simulink model "ProvaSCADA"  (R2024b)
settings: Solver=FixedStepAuto  StartTime=0.0  StopTime=Tsim  FixedStep=dT  RelTol=1e-3
values from neighbouring files (symbols this model uses):
  b = t + 2*s    (= 3.6)    [ParametriSegheria.m]    (also in ParametriSegheriaDinamica.m)
  h_index = [70, 80, 90, 100]    [ParametriSegheria.m]    (also in ParametriSegheriaDinamica.m)
  J1 = 8*1e6    (= 8000000)    [ParametriSegheriaDinamica.m]
  J2 = 0.9*1e6    (= 900000)    [ParametriSegheriaDinamica.m]
  kc = [0 35 40 50 55 90]    [ParametriSegheria.m]    (also in ParametriSegheriaDinamica.m = [0, 25, 30, 35, 50, 70])
  Kt = 2    [ParametriSegheria.m]    (also in ParametriSegheriaDinamica.m = 10000)
  Kt2 = 5    [ParametriSegheria.m]    (also in ParametriSegheriaDinamica.m = 4500)
  l_index = [20, 30, 40, 50]    [ParametriSegheria.m]    (also in ParametriSegheriaDinamica.m)
  Lt = 4    [ParametriSegheria.m]    (also in ParametriSegheriaDinamica.m)
  Mag_D = [0 430 320 260 230 540 430 320 260 230 540 430 320 260 230 540 430 320 260 230 540 430 320 260 230 540 430 320 260 230 540]    [ParametriSegheria.m]    (also in ParametriSegheriaDinamica.m = [0 randi([220 500], 1, 150)])
  Mag_legno = [0 1 5 2 4 3 1 5 2 4 3 1 5 2 4 3 1 5 2 4 3 1 5 2 4 3 1 5 2 4 3]    [ParametriSegheria.m]    (also in ParametriSegheriaDinamica.m = [0 randi([1 5], 1, 150)])
  n_sottili = 4    [ParametriSegheria.m]    (also in ParametriSegheriaDinamica.m)
  omega_ref1 = 50    [ParametriSegheriaDinamica.m]
  omega_ref2 = 3000*(2*pi/60)    (= 314.159265359)    [ParametriSegheriaDinamica.m]
  Rc = 200    [ParametriSegheria.m]    (also in ParametriSegheriaDinamica.m)
  rho = [0, 450, 520, 590, 710, 780]*1e-9    [ParametriSegheriaDinamica.m]
  Rs = 800    [ParametriSegheria.m]    (also in ParametriSegheriaDinamica.m)
  SR = Rs/Rm    (= 5.33333333333)    [ParametriSegheria.m]    (also in ParametriSegheriaDinamica.m)
  SR2 = Rc/Rm2    (= 4)    [ParametriSegheria.m]    (also in ParametriSegheriaDinamica.m)
undefined symbols (not defined in the file or in its folder): thrsh
libraries: simulink x6, slpidlib x6
(part 1 of 2)
settings Model: Creator=samue  LastModifiedBy=samue

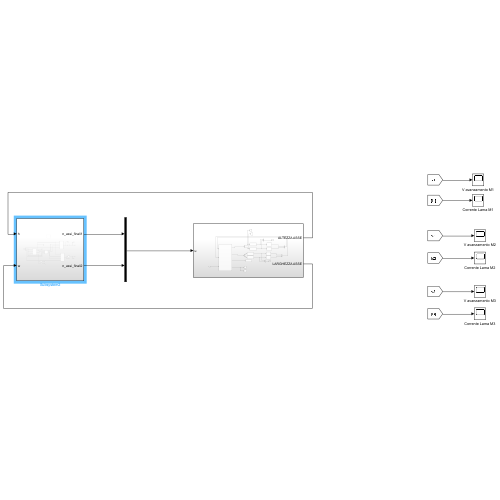
[thumbnail: Simulink's stored preview of the top-level diagram]
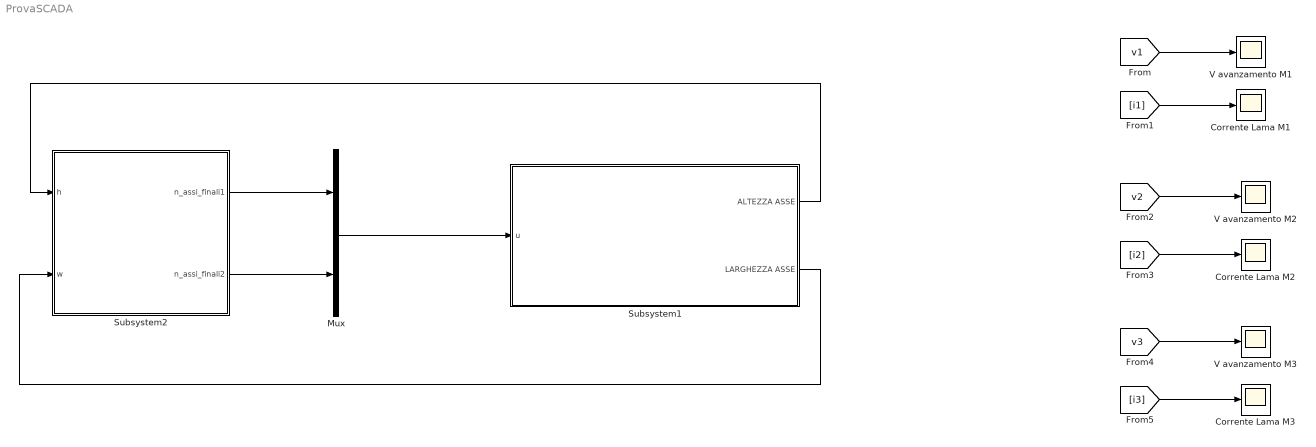
== system ProvaSCADA ==
  Corrente Lama M1 : Scope
  Corrente Lama M2 : Scope
  Corrente Lama M3 : Scope
  Mux : Mux  Inputs=2
  Subsystem1 : Subsystem
  Subsystem2 : Subsystem
  V avanzamento M1 : Scope
  V avanzamento M2 : Scope
  V avanzamento M3 : Scope
  wires:
  Subsystem2/2(n_assi_finali2) -> Mux/2
  [i3] -> Corrente Lama M3/1
  [i1] -> Corrente Lama M1/1
  [i2] -> Corrente Lama M2/1
  Subsystem2/1(n_assi_finali1) -> Mux/1
  [v2] -> V avanzamento M2/1
  [v1] -> V avanzamento M1/1
  [v3] -> V avanzamento M3/1
  Mux/1 -> Subsystem1/1(u)
  Subsystem1/1(ALTEZZA ASSE) -> Subsystem2/1(h)
  Subsystem1/2(LARGHEZZA ASSE) -> Subsystem2/2(w)

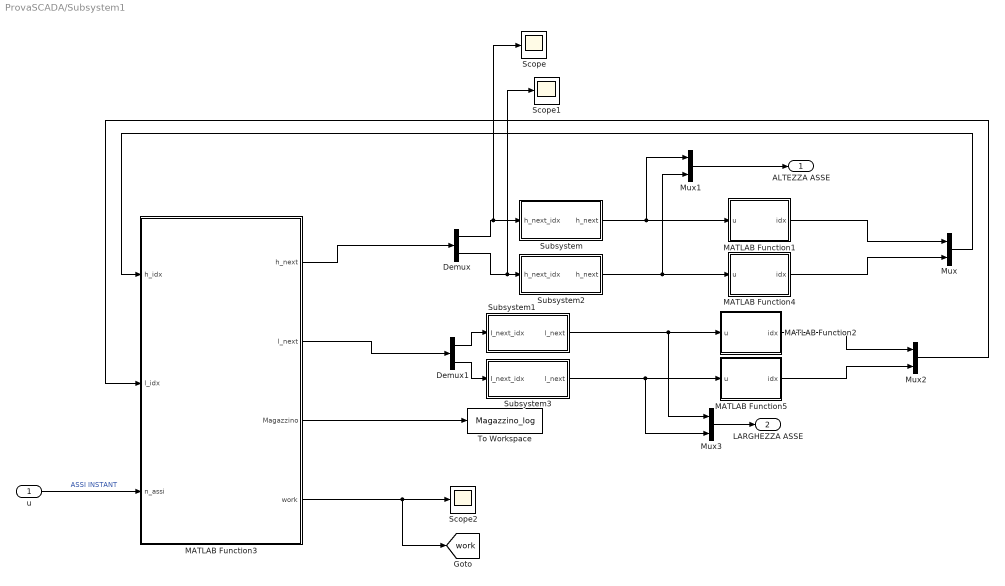
== system ProvaSCADA/Subsystem1 ==
  u : Inport
  Demux : Demux  Outputs=2
  Demux1 : Demux  Outputs=2
  MATLAB Function1 : MATLAB Function  TreatAsAtomicUnit=on
  MATLAB Function2 : MATLAB Function  TreatAsAtomicUnit=on
  MATLAB Function3 : MATLAB Function  TreatAsAtomicUnit=on
  MATLAB Function4 : MATLAB Function  TreatAsAtomicUnit=on
  MATLAB Function5 : MATLAB Function  TreatAsAtomicUnit=on
  Mux{,1..3} (4 alike) : Mux  Inputs=2
  Scope : Scope
  Scope1 : Scope
  Scope2 : Scope
  Subsystem : Subsystem
  Subsystem1 : Subsystem
  Subsystem2 : Subsystem
  Subsystem3 : Subsystem
  To Workspace : ToWorkspace  VariableName=Magazzino_log  SaveFormat=Timeseries  SampleTime=-1
  ALTEZZA ASSE : Outport
  LARGHEZZA ASSE : Outport  Port=2
  tag scope: work=global
  wires:
  MATLAB Function3/3(Magazzino) -> To Workspace/1
  u/1 -> MATLAB Function3/3(n_assi)  "ASSI INSTANT"
  Subsystem/1(h_next) -> Mux1/1, MATLAB Function1/1(u)
  Subsystem1/1(l_next) -> Mux3/1, MATLAB Function2/1(u)
  MATLAB Function3/1(h_next) -> Demux/1
  Subsystem2/1(h_next) -> Mux1/2, MATLAB Function4/1(u)
  Demux/2 -> Scope1/1, Subsystem2/1(h_next_idx)
  Demux/1 -> Scope/1, Subsystem/1(h_next_idx)
  MATLAB Function1/1(idx) -> Mux/1
  MATLAB Function4/1(idx) -> Mux/2
  Mux/1 -> MATLAB Function3/1(h_idx)
  Mux1/1 -> ALTEZZA ASSE/1
  Subsystem3/1(l_next) -> Mux3/2, MATLAB Function5/1(u)
  MATLAB Function3/2(l_next) -> Demux1/1
  Demux1/1 -> Subsystem1/1(I_next_idx)
  Demux1/2 -> Subsystem3/1(I_next_idx)
  Mux3/1 -> LARGHEZZA ASSE/1
  MATLAB Function2/1(idx) -> Mux2/1
  MATLAB Function5/1(idx) -> Mux2/2
  Mux2/1 -> MATLAB Function3/2(l_idx)
  MATLAB Function3/4(work) -> [work], Scope2/1

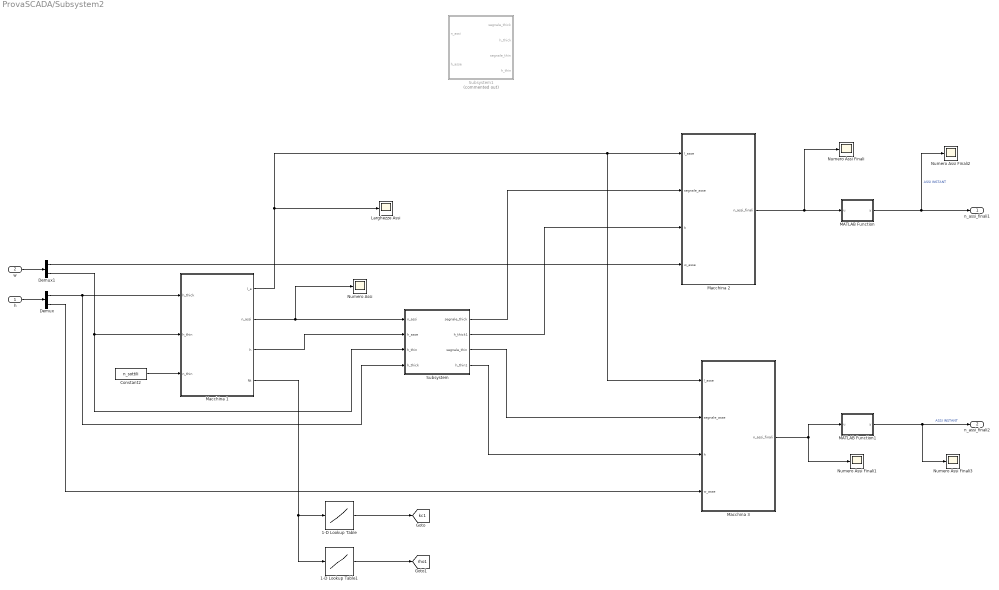
== system ProvaSCADA/Subsystem2 ==
  h : Inport
  w : Inport  Port=2
  1-D Lookup Table : Lookup_n-D  NumberOfTableDimensions=1  BreakpointsForDimension1=[0 1 2 3 4 5 ]  Table=kc  InternalRulePriority=Speed  RndMeth=Simplest
  1-D Lookup Table1 : Lookup_n-D  NumberOfTableDimensions=1  BreakpointsForDimension1=[0 1 2 3 4 5 ]  Table=rho  InternalRulePriority=Speed  RndMeth=Simplest
  Constant2 : Constant  Value=n_sottili
  Demux : Demux  Outputs=2
  Demux1 : Demux  Outputs=2
  Larghezze Assi : Scope
  MATLAB Function : MATLAB Function  TreatAsAtomicUnit=on
  MATLAB Function1 : MATLAB Function  TreatAsAtomicUnit=on
  Macchina 1 : Subsystem
  Macchina 2 : Subsystem
  Macchina 3 : Subsystem
  Numero Assi : Scope
  Numero Assi Finali{,1..3} (4 alike) : Scope
  Subsystem : Subsystem
  Subsystem1 : Subsystem  Commented=on
  n_assi_finali1 : Outport
  n_assi_finali2 : Outport  Port=2
  tag scope: kc1=global, rho1=global
  wires:
  Macchina 1/1(l_a) -> Larghezze Assi/1, Macchina 3/1(l_asse), Macchina 2/1(l_asse)
  Macchina 1/2(n_assi) -> Numero Assi/1, Subsystem/1(n_assi)
  Macchina 1/3(h) -> Subsystem/2(h_asse)
  Constant2/1 -> Macchina 1/3(n_thin)
  Macchina 3/1(n_assi_finali) -> Numero Assi Finali1/1, MATLAB Function1/1(u)
  Macchina 2/1(n_assi_finali) -> Numero Assi Finali/1, MATLAB Function/1(u)
  MATLAB Function/1(y) -> Numero Assi Finali2/1, n_assi_finali1/1  "ASSI INSTANT"
  MATLAB Function1/1(y) -> Numero Assi Finali3/1, n_assi_finali2/1  "ASSI INSTANT"
  Subsystem/1(segnale_thick) -> Macchina 2/2(segnale_asse)
  Subsystem/2(h_thick1) -> Macchina 2/3(h)
  Subsystem/3(segnale_thin) -> Macchina 3/2(segnale_asse)
  Subsystem/4(h_thin1) -> Macchina 3/3(h)
  1-D Lookup Table/1 -> [kc1]
  1-D Lookup Table1/1 -> [rho1]
  Macchina 1/4(Nt) -> 1-D Lookup Table1/1, 1-D Lookup Table/1
  h/1 -> Demux/1
  w/1 -> Demux1/1
  Demux/2 -> Macchina 3/4(w_asse)
  Demux/1 -> Macchina 1/1(h_thick), Subsystem/4(h_thick)
  Demux1/1 -> Macchina 2/4(w_asse)
  Demux1/2 -> Subsystem/3(h_thin), Macchina 1/2(h_thin)

== system ProvaSCADA/Subsystem1/Subsystem ==
  h_next_idx : Inport
  Constant4 : Constant  Value=h_index
  Constant7 : Constant
  Memory : Memory
  SELEZIONE ALTEZZA : Selector  InputPortWidth=length(h_index)  IndexOptions=Index vector (port)  Indices=[1 3]  OutputSizes=1
  Switch1 : Switch  Criteria=u2 > Threshold  SaturateOnIntegerOverflow=off  InputSameDT=off
  h_next : Outport
  wires:
  h_next_idx/1 -> Memory/1
  Constant7/1 -> Switch1/3
  Memory/1 -> Switch1/2, Switch1/1
  SELEZIONE ALTEZZA/1 -> h_next/1
  Constant4/1 -> SELEZIONE ALTEZZA/1
  Switch1/1 -> SELEZIONE ALTEZZA/2

== system ProvaSCADA/Subsystem1/Subsystem1 ==
  I_next_idx : Inport
  Constant5 : Constant  Value=l_index
  Constant8 : Constant
  Memory1 : Memory
  SELEZIONE LUNGHEZZA : Selector  InputPortWidth=length(h_index)  IndexOptions=Index vector (port)  Indices=[1 3]  OutputSizes=1
  Switch2 : Switch  Criteria=u2 > Threshold  SaturateOnIntegerOverflow=off  InputSameDT=off
  l_next : Outport
  wires:
  Memory1/1 -> Switch2/1, Switch2/2
  SELEZIONE LUNGHEZZA/1 -> l_next/1
  Switch2/1 -> SELEZIONE LUNGHEZZA/2
  Constant5/1 -> SELEZIONE LUNGHEZZA/1
  I_next_idx/1 -> Memory1/1
  Constant8/1 -> Switch2/3

== system ProvaSCADA/Subsystem1/Subsystem2 ==
  h_next_idx : Inport
  Constant4 : Constant  Value=h_index
  Constant7 : Constant
  Memory : Memory
  SELEZIONE ALTEZZA : Selector  InputPortWidth=length(h_index)  IndexOptions=Index vector (port)  Indices=[1 3]  OutputSizes=1
  Switch1 : Switch  Criteria=u2 > Threshold  SaturateOnIntegerOverflow=off  InputSameDT=off
  h_next : Outport
  wires:
  Switch1/1 -> SELEZIONE ALTEZZA/2
  Constant4/1 -> SELEZIONE ALTEZZA/1
  SELEZIONE ALTEZZA/1 -> h_next/1
  Memory/1 -> Switch1/1, Switch1/2
  Constant7/1 -> Switch1/3
  h_next_idx/1 -> Memory/1

== system ProvaSCADA/Subsystem1/Subsystem3 ==
  I_next_idx : Inport
  Constant5 : Constant  Value=l_index
  Constant8 : Constant
  Memory1 : Memory
  SELEZIONE LUNGHEZZA : Selector  InputPortWidth=length(h_index)  IndexOptions=Index vector (port)  Indices=[1 3]  OutputSizes=1
  Switch2 : Switch  Criteria=u2 > Threshold  SaturateOnIntegerOverflow=off  InputSameDT=off
  l_next : Outport
  wires:
  Constant8/1 -> Switch2/3
  I_next_idx/1 -> Memory1/1
  Constant5/1 -> SELEZIONE LUNGHEZZA/1
  Switch2/1 -> SELEZIONE LUNGHEZZA/2
  SELEZIONE LUNGHEZZA/1 -> l_next/1
  Memory1/1 -> Switch2/2, Switch2/1

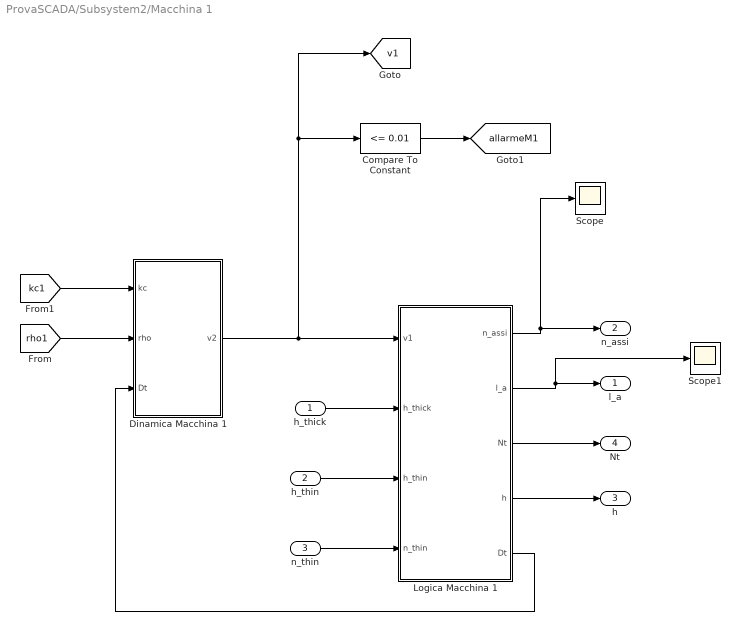
== system ProvaSCADA/Subsystem2/Macchina 1 ==
  h_thick : Inport
  h_thin : Inport  Port=2
  n_thin : Inport  Port=3
  Compare To Constant : simulink/Logic and Bit Operations/Compare To Constant  relop=<=  const=0.01  OutDataTypeStr=boolean
  Dinamica Macchina 1 : Subsystem
  Logica Macchina 1 : Subsystem
  Scope : Scope
  Scope1 : Scope
  l_a : Outport
  n_assi : Outport  Port=2
  h : Outport  Port=3
  Nt : Outport  Port=4
  tag scope: allarmeM1=global, v1=global
  wires:
  Dinamica Macchina 1/1(v2) -> Compare To Constant/1, [v1], Logica Macchina 1/1(v1)
  Logica Macchina 1/3(Nt) -> Nt/1
  Logica Macchina 1/1(n_assi) -> Scope/1, n_assi/1
  Logica Macchina 1/2(l_a) -> Scope1/1, l_a/1
  h_thick/1 -> Logica Macchina 1/2(h_thick)
  h_thin/1 -> Logica Macchina 1/3(h_thin)
  n_thin/1 -> Logica Macchina 1/4(n_thin)
  Logica Macchina 1/4(h) -> h/1
  [rho1] -> Dinamica Macchina 1/2(rho)
  [kc1] -> Dinamica Macchina 1/1(kc)
  Logica Macchina 1/5(Dt) -> Dinamica Macchina 1/3(Dt)
  Compare To Constant/1 -> [allarmeM1]

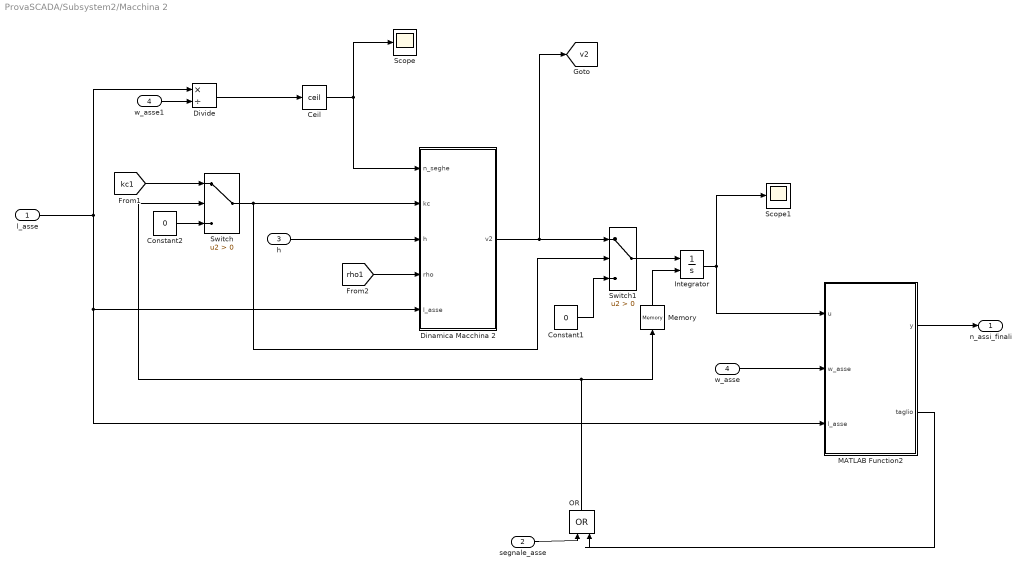
== system ProvaSCADA/Subsystem2/Macchina 2 ==
  l_asse : Inport
  segnale_asse : Inport  Port=2
  h : Inport  Port=3
  w_asse : Inport  Port=4
  Ceil : Rounding  Operator=ceil
  Constant1 : Constant  Value=0
  Constant2 : Constant  Value=0
  Dinamica Macchina 2 : Subsystem
  Divide : Product  Inputs=*/
  Integrator : Integrator  ExternalReset=falling
  MATLAB Function2 : MATLAB Function  TreatAsAtomicUnit=on
  Memory : Memory
  OR : Logic  Operator=OR  IconShape=distinctive  AllPortsSameDT=off  OutDataTypeStr=boolean
  Scope : Scope
  Scope1 : Scope
  Switch : Switch  Criteria=u2 > Threshold  SaturateOnIntegerOverflow=off  InputSameDT=off
  Switch1 : Switch  Criteria=u2 > Threshold  SaturateOnIntegerOverflow=off  InputSameDT=off
  w_asse1 : InportShadow  Port=4
  n_assi_finali : Outport
  tag scope: v2=global
  wires:
  Divide/1 -> Ceil/1
  OR/1 -> Switch/2, Memory/1
  Dinamica Macchina 2/1(v2) -> Switch1/1, [v2]
  Constant2/1 -> Switch/3
  Switch/1 -> Dinamica Macchina 2/2(kc), Switch1/2
  Integrator/1 -> MATLAB Function2/1(u), Scope1/1
  MATLAB Function2/2(taglio) -> OR/2
  h/1 -> Dinamica Macchina 2/3(h)
  l_asse/1 -> MATLAB Function2/3(l_asse), Dinamica Macchina 2/5(l_asse), Divide/1
  Ceil/1 -> Scope/1, Dinamica Macchina 2/1(n_seghe)
  Memory/1 -> Integrator/2
  [kc1] -> Switch/1
  w_asse1/1 -> Divide/2
  segnale_asse/1 -> OR/1
  w_asse/1 -> MATLAB Function2/2(w_asse)
  [rho1] -> Dinamica Macchina 2/4(rho)
  Switch1/1 -> Integrator/1
  Constant1/1 -> Switch1/3
  MATLAB Function2/1(y) -> n_assi_finali/1

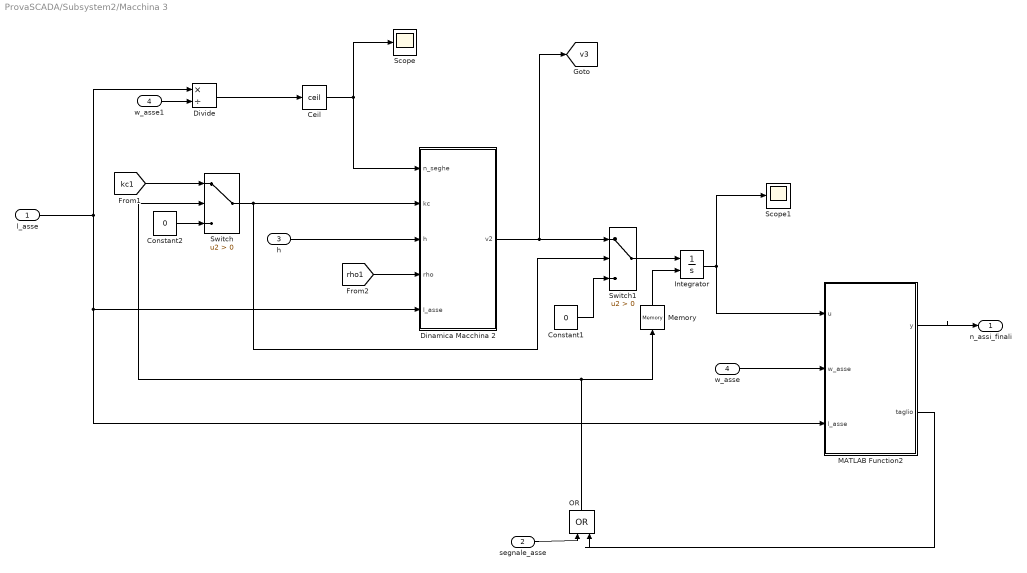
== system ProvaSCADA/Subsystem2/Macchina 3 ==
  l_asse : Inport
  segnale_asse : Inport  Port=2
  h : Inport  Port=3
  w_asse : Inport  Port=4
  Ceil : Rounding  Operator=ceil
  Constant1 : Constant  Value=0
  Constant2 : Constant  Value=0
  Dinamica Macchina 2 : Subsystem
  Divide : Product  Inputs=*/
  Integrator : Integrator  ExternalReset=falling
  MATLAB Function2 : MATLAB Function  TreatAsAtomicUnit=on
  Memory : Memory
  OR : Logic  Operator=OR  IconShape=distinctive  AllPortsSameDT=off  OutDataTypeStr=boolean
  Scope : Scope
  Scope1 : Scope
  Switch : Switch  Criteria=u2 > Threshold  SaturateOnIntegerOverflow=off  InputSameDT=off
  Switch1 : Switch  Criteria=u2 > Threshold  SaturateOnIntegerOverflow=off  InputSameDT=off
  w_asse1 : InportShadow  Port=4
  n_assi_finali : Outport
  tag scope: v3=global
  wires:
  Divide/1 -> Ceil/1
  OR/1 -> Switch/2, Memory/1
  Dinamica Macchina 2/1(v2) -> Switch1/1, [v3]
  Constant2/1 -> Switch/3
  Switch/1 -> Dinamica Macchina 2/2(kc), Switch1/2
  Integrator/1 -> MATLAB Function2/1(u), Scope1/1
  MATLAB Function2/2(taglio) -> OR/2
  h/1 -> Dinamica Macchina 2/3(h)
  l_asse/1 -> MATLAB Function2/3(l_asse), Dinamica Macchina 2/5(l_asse), Divide/1
  Ceil/1 -> Scope/1, Dinamica Macchina 2/1(n_seghe)
  Memory/1 -> Integrator/2
  [kc1] -> Switch/1
  MATLAB Function2/1(y) -> n_assi_finali/1
  w_asse1/1 -> Divide/2
  segnale_asse/1 -> OR/1
  w_asse/1 -> MATLAB Function2/2(w_asse)
  [rho1] -> Dinamica Macchina 2/4(rho)
  Switch1/1 -> Integrator/1
  Constant1/1 -> Switch1/3

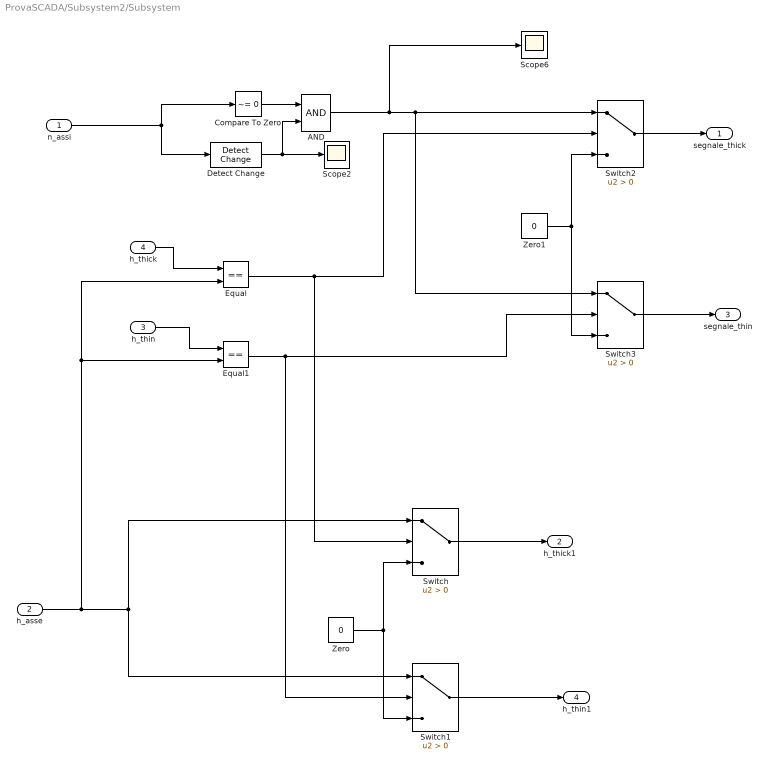
== system ProvaSCADA/Subsystem2/Subsystem ==
  n_assi : Inport
  h_asse : Inport  Port=2
  h_thin : Inport  Port=3
  h_thick : Inport  Port=4
  AND : Logic  IconShape=distinctive  AllPortsSameDT=off  OutDataTypeStr=boolean
  Compare To Zero : simulink/Logic and Bit Operations/Compare To Zero  relop=~=  OutDataTypeStr=boolean
  Detect Change : simulink/Logic and Bit Operations/Detect Change  vinit=0  OutDataTypeStr=boolean
  Equal : RelationalOperator  Operator===  OutDataTypeStr=boolean  RndMeth=Simplest  InputSameDT=off
  Equal1 : RelationalOperator  Operator===  OutDataTypeStr=boolean  RndMeth=Simplest  InputSameDT=off
  Scope2 : Scope
  Scope6 : Scope
  Switch{,1..3} (4 alike) : Switch  Criteria=u2 > Threshold  SaturateOnIntegerOverflow=off  InputSameDT=off
  Zero : Constant  Value=0  OutDataTypeStr=Inherit: Inherit via back propagation
  Zero1 : Constant  Value=0  OutDataTypeStr=Inherit: Inherit via back propagation
  segnale_thick : Outport
  h_thick1 : Outport  Port=2
  segnale_thin : Outport  Port=3
  h_thin1 : Outport  Port=4
  wires:
  Detect Change/1 -> Scope2/1, AND/2
  Zero/1 -> Switch/3, Switch1/3
  Switch/1 -> h_thick1/1
  n_assi/1 -> Compare To Zero/1, Detect Change/1
  Compare To Zero/1 -> AND/1
  Switch1/1 -> h_thin1/1
  Zero1/1 -> Switch2/3, Switch3/3
  h_asse/1 -> Equal1/2, Equal/2, Switch/1, Switch1/1
  Switch2/1 -> segnale_thick/1
  AND/1 -> Switch3/1, Switch2/1, Scope6/1
  Switch3/1 -> segnale_thin/1
  h_thick/1 -> Equal/1
  Equal/1 -> Switch/2, Switch2/2
  h_thin/1 -> Equal1/1
  Equal1/1 -> Switch1/2, Switch3/2

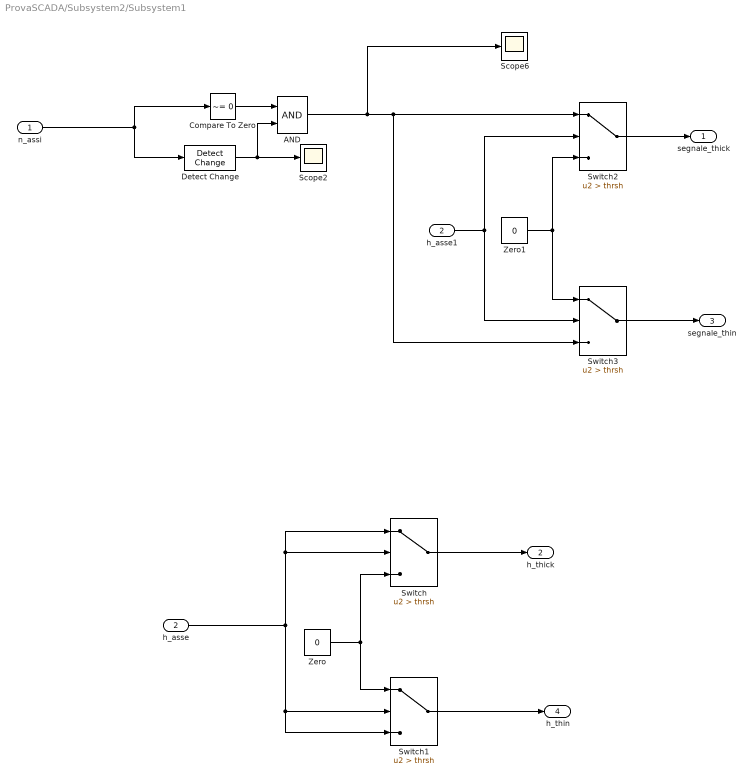
== system ProvaSCADA/Subsystem2/Subsystem1 ==
  n_assi : Inport
  h_asse : Inport  Port=2
  AND : Logic  IconShape=distinctive  AllPortsSameDT=off  OutDataTypeStr=boolean
  Compare To Zero : simulink/Logic and Bit Operations/Compare To Zero  relop=~=  OutDataTypeStr=boolean
  Detect Change : simulink/Logic and Bit Operations/Detect Change  vinit=0  OutDataTypeStr=boolean
  Scope2 : Scope
  Scope6 : Scope
  Switch{,1..3} (4 alike) : Switch  Criteria=u2 > Threshold  Threshold=thrsh  SaturateOnIntegerOverflow=off  InputSameDT=off
  Zero : Constant  Value=0  OutDataTypeStr=Inherit: Inherit via back propagation
  Zero1 : Constant  Value=0  OutDataTypeStr=Inherit: Inherit via back propagation
  h_asse1 : InportShadow  Port=2
  segnale_thick : Outport
  h_thick : Outport  Port=2
  segnale_thin : Outport  Port=3
  h_thin : Outport  Port=4
  wires:
  Detect Change/1 -> Scope2/1, AND/2
  Zero/1 -> Switch1/1, Switch/3
  Switch/1 -> h_thick/1
  n_assi/1 -> Compare To Zero/1, Detect Change/1
  Compare To Zero/1 -> AND/1
  Switch1/1 -> h_thin/1
  Zero1/1 -> Switch2/3, Switch3/1
  h_asse/1 -> Switch/1, Switch/2, Switch1/2, Switch1/3
  Switch2/1 -> segnale_thick/1
  h_asse1/1 -> Switch2/2, Switch3/2
  AND/1 -> Switch3/3, Switch2/1, Scope6/1
  Switch3/1 -> segnale_thin/1

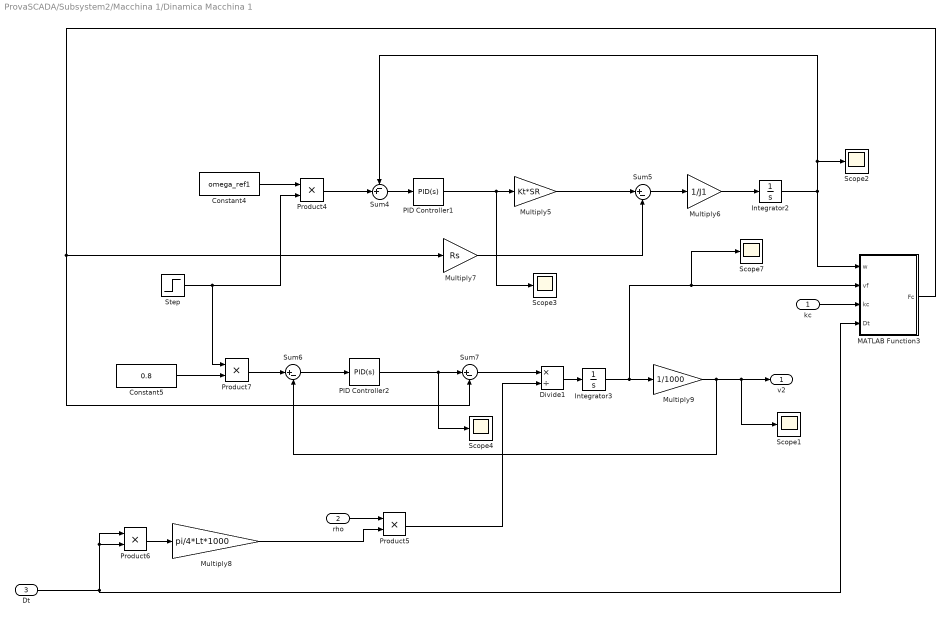
== system ProvaSCADA/Subsystem2/Macchina 1/Dinamica Macchina 1 ==
  kc : Inport
  rho : Inport  Port=2
  Dt : Inport  Port=3
  Constant4 : Constant  Value=omega_ref1
  Constant5 : Constant  Value=0.8
  Divide1 : Product  Inputs=*/
  Integrator2 : Integrator  InitialCondition=omega_ref1
  Integrator3 : Integrator  InitialCondition=800
  MATLAB Function3 : MATLAB Function  TreatAsAtomicUnit=on
  Multiply5 : Gain  Gain=Kt*SR
  Multiply6 : Gain  Gain=1/J1
  Multiply7 : Gain  Gain=Rs
  Multiply8 : Gain  Gain=pi/4*Lt*1000
  Multiply9 : Gain  Gain=1/1000
  PID Controller1 : slpidlib/PID Controller  Controller=PID  Form=Parallel  TimeDomain=Continuous-time  UseExternalTs=off  SampleTime=-1  IntegratorMethod=Forward Euler  FilterMethod=Forward Euler  ControllerParametersSource=internal  P=1298.12673021629  I=2057.42177441043  UseKiTs=off  D=19.7220789716769  UseExternalDerivativeSource=off  N=48.3817350429841  UseFilter=on  TunerSelectOption=Transfer Function Based (PID Tuner App)  InitialConditionSource=internal  InitialConditionForIntegrator=0  InitialConditionForFilter=0  DifferentiatorICPrevScaledInput=0  ExternalReset=none  TrackingMode=off  Kt=1  LimitOutput=on  SatLimitsSource=internal  UpperSaturationLimit=300  LowerSaturationLimit=-300  LinearizeAsGain=off  AntiWindupMode=clamping  Kb=1  LimitIntegrator=off  UpperIntegratorSaturationLimit=200  LowerIntegratorSaturationLimit=-inf  POutMin=[]  POutMax=[]  IOutMin=[]  IOutMax=[]  DOutMin=[]  DOutMax=[]  NOutMin=[]  NOutMax=[]  SumOutMin=[]  SumOutMax=[]  SaturationOutMin=[]  SaturationOutMax=[]  PParamMin=[]  PParamMax=[]  IParamMin=[]  IParamMax=[]  DParamMin=[]  DParamMax=[]  NParamMin=[]  NParamMax=[]  KbParamMin=[]  KbParamMax=[]  KtParamMin=[]  KtParamMax=[]  KbOutMin=[]  KbOutMax=[]  KtOutMin=[]  KtOutMax=[]  IntegratorOutMin=[]  IntegratorOutMax=[]  FilterOutMin=[]  FilterOutMax=[]  SumI1OutMin=[]  SumI1OutMax=[]  SumI2OutMin=[]  SumI2OutMax=[]  SumI3OutMin=[]  SumI3OutMax=[]  SumI4OutMin=[]  SumI4OutMax=[]  SumDOutMin=[]  SumDOutMax=[]  DifferentiatorOutMin=[]  DifferentiatorOutMax=[]  FilterDiffOutCoefMin=[]  FilterDiffOutCoefMax=[]  ReciprocalOutMin=[]  ReciprocalOutMax=[]  SumDenOutMin=[]  SumDenOutMax=[]  SumNumOutMin=[]  SumNumOutMax=[]  DivideOutMin=[]  DivideOutMax=[]  UdiffTsProdOutMin=[]  UdiffTsProdOutMax=[]  NTsProdOutMin=[]  NTsProdOutMax=[]  UintegralTsProdOutMin=[]  UintegralTsProdOutMax=[]  UngainTsProdOutMin=[]  UngainTsProdOutMax=[]  ClampingZeroOutDataTypeStr=Inherit: Inherit via back propagation  ClampingZeroOutMin=[]  ClampingZeroOutMax=[]  FilterDenConstantOutDataTypeStr=Inherit: Inherit via back propagation  FilterDenConstantOutMin=[]  FilterDenConstantOutMax=[]  PCopyOutDataTypeStr=Inherit: Inherit via back propagation  PCopyOutMin=[]  PCopyOutMax=[]  NCopyOutDataTypeStr=Inherit: Inherit via back propagation  NCopyOutMin=[]  NCopyOutMax=[]  IntegratorContinuousStateAttributes=''  IntegratorStateMustResolveToSignalObject=off  IntegratorRTWStateStorageClass=Auto  FilterContinuousStateAttributes=''  FilterStateMustResolveToSignalObject=off  FilterRTWStateStorageClass=Auto  ParallelPVariant=InternalParameters  IdealPVariant=Disabled  IVariant=InternalParameters  DVariant=InternalParameters  IntegratorVariant=Continuous  SatVariant=Enabled  AWVariant=ContClampingParallel  PCopyVariant=Disabled  TRVariant=Disabled  FdbkBlocksVariant=Forward  IdealPFdbkVariant=Disabled  SatFdbkVariant=Disabled  DerivativeFilterVariant=ContFilter  NVariant=InternalParameters  NCopyVariant=Disabled  FilterICVariant=InternalICsFilter  IntegratorICVariant=InternalICs  ExternalResetVariant=Disabled  TRSumVariant=Passthrough  SumFdbkVariant=Disabled  SumVariant=Sum_PID  TsampFilterVariant=InternalTs  TsampNgainVariant=Passthrough  TsampIntegralVariant=Disabled_SignalSpec  ExternalSaturationOutDataTypeStr=Inherit: Same as second input  DerivativeSourceVariant=ErrorSignal  PreIntVariant=InternalPreInt
  PID Controller2 : slpidlib/PID Controller  Controller=PID  Form=Parallel  TimeDomain=Continuous-time  UseExternalTs=off  SampleTime=-1  IntegratorMethod=Forward Euler  FilterMethod=Forward Euler  ControllerParametersSource=internal  P=1286337.49585534  I=1467032.44527875  UseKiTs=off  D=37575.4377581997  UseExternalDerivativeSource=off  N=23.5405770451102  UseFilter=on  TunerSelectOption=Transfer Function Based (PID Tuner App)  InitialConditionSource=internal  InitialConditionForIntegrator=0  InitialConditionForFilter=0  DifferentiatorICPrevScaledInput=0  ExternalReset=none  TrackingMode=off  Kt=1  LimitOutput=on  SatLimitsSource=internal  UpperSaturationLimit=6000  LowerSaturationLimit=-6000  LinearizeAsGain=off  AntiWindupMode=clamping  Kb=1  LimitIntegrator=off  UpperIntegratorSaturationLimit=200  LowerIntegratorSaturationLimit=-inf  POutMin=[]  POutMax=[]  IOutMin=[]  IOutMax=[]  DOutMin=[]  DOutMax=[]  NOutMin=[]  NOutMax=[]  SumOutMin=[]  SumOutMax=[]  SaturationOutMin=[]  SaturationOutMax=[]  PParamMin=[]  PParamMax=[]  IParamMin=[]  IParamMax=[]  DParamMin=[]  DParamMax=[]  NParamMin=[]  NParamMax=[]  KbParamMin=[]  KbParamMax=[]  KtParamMin=[]  KtParamMax=[]  KbOutMin=[]  KbOutMax=[]  KtOutMin=[]  KtOutMax=[]  IntegratorOutMin=[]  IntegratorOutMax=[]  FilterOutMin=[]  FilterOutMax=[]  SumI1OutMin=[]  SumI1OutMax=[]  SumI2OutMin=[]  SumI2OutMax=[]  SumI3OutMin=[]  SumI3OutMax=[]  SumI4OutMin=[]  SumI4OutMax=[]  SumDOutMin=[]  SumDOutMax=[]  DifferentiatorOutMin=[]  DifferentiatorOutMax=[]  FilterDiffOutCoefMin=[]  FilterDiffOutCoefMax=[]  ReciprocalOutMin=[]  ReciprocalOutMax=[]  SumDenOutMin=[]  SumDenOutMax=[]  SumNumOutMin=[]  SumNumOutMax=[]  DivideOutMin=[]  DivideOutMax=[]  UdiffTsProdOutMin=[]  UdiffTsProdOutMax=[]  NTsProdOutMin=[]  NTsProdOutMax=[]  UintegralTsProdOutMin=[]  UintegralTsProdOutMax=[]  UngainTsProdOutMin=[]  UngainTsProdOutMax=[]  ClampingZeroOutDataTypeStr=Inherit: Inherit via back propagation  ClampingZeroOutMin=[]  ClampingZeroOutMax=[]  FilterDenConstantOutDataTypeStr=Inherit: Inherit via back propagation  FilterDenConstantOutMin=[]  FilterDenConstantOutMax=[]  PCopyOutDataTypeStr=Inherit: Inherit via back propagation  PCopyOutMin=[]  PCopyOutMax=[]  NCopyOutDataTypeStr=Inherit: Inherit via back propagation  NCopyOutMin=[]  NCopyOutMax=[]  IntegratorContinuousStateAttributes=''  IntegratorStateMustResolveToSignalObject=off  IntegratorRTWStateStorageClass=Auto  FilterContinuousStateAttributes=''  FilterStateMustResolveToSignalObject=off  FilterRTWStateStorageClass=Auto  ParallelPVariant=InternalParameters  IdealPVariant=Disabled  IVariant=InternalParameters  DVariant=InternalParameters  IntegratorVariant=Continuous  SatVariant=Enabled  AWVariant=ContClampingParallel  PCopyVariant=Disabled  TRVariant=Disabled  FdbkBlocksVariant=Forward  IdealPFdbkVariant=Disabled  SatFdbkVariant=Disabled  DerivativeFilterVariant=ContFilter  NVariant=InternalParameters  NCopyVariant=Disabled  FilterICVariant=InternalICsFilter  IntegratorICVariant=InternalICs  ExternalResetVariant=Disabled  TRSumVariant=Passthrough  SumFdbkVariant=Disabled  SumVariant=Sum_PID  TsampFilterVariant=InternalTs  TsampNgainVariant=Passthrough  TsampIntegralVariant=Disabled_SignalSpec  ExternalSaturationOutDataTypeStr=Inherit: Same as second input  DerivativeSourceVariant=ErrorSignal  PreIntVariant=InternalPreInt
  Product{4..7} (4 alike) : Product
  Scope{1..4,7} (5 alike) : Scope
  Step : Step  Time=5000  Before=1  After=0  SampleTime=0
  Sum4 : Sum  Inputs=-+|
  Sum5 : Sum  Inputs=|+-
  Sum6 : Sum  Inputs=|+-
  Sum7 : Sum  Inputs=|+-
  v2 : Outport
  wires:
  Constant4/1 -> Product4/1
  Constant5/1 -> Product7/2
  Product5/1 -> Divide1/2
  Product4/1 -> Sum4/2
  Sum4/1 -> PID Controller1/1
  Step/1 -> Product4/2, Product7/1
  Product6/1 -> Multiply8/1
  Sum5/1 -> Multiply6/1
  kc/1 -> MATLAB Function3/3(kc)
  Multiply6/1 -> Integrator2/1
  PID Controller1/1 -> Scope3/1, Multiply5/1
  Multiply8/1 -> Product5/2
  MATLAB Function3/1(Fc) -> Sum7/2, Multiply7/1
  Sum6/1 -> PID Controller2/1
  Dt/1 -> Product6/1, Product6/2, MATLAB Function3/4(Dt)
  Divide1/1 -> Integrator3/1
  Integrator3/1 -> Scope7/1, MATLAB Function3/2(vf), Multiply9/1
  Multiply9/1 -> Scope1/1, v2/1, Sum6/2
  Integrator2/1 -> MATLAB Function3/1(w), Scope2/1, Sum4/1
  Sum7/1 -> Divide1/1
  Product7/1 -> Sum6/1
  rho/1 -> Product5/1
  PID Controller2/1 -> Scope4/1, Sum7/1
  Multiply5/1 -> Sum5/1
  Multiply7/1 -> Sum5/2

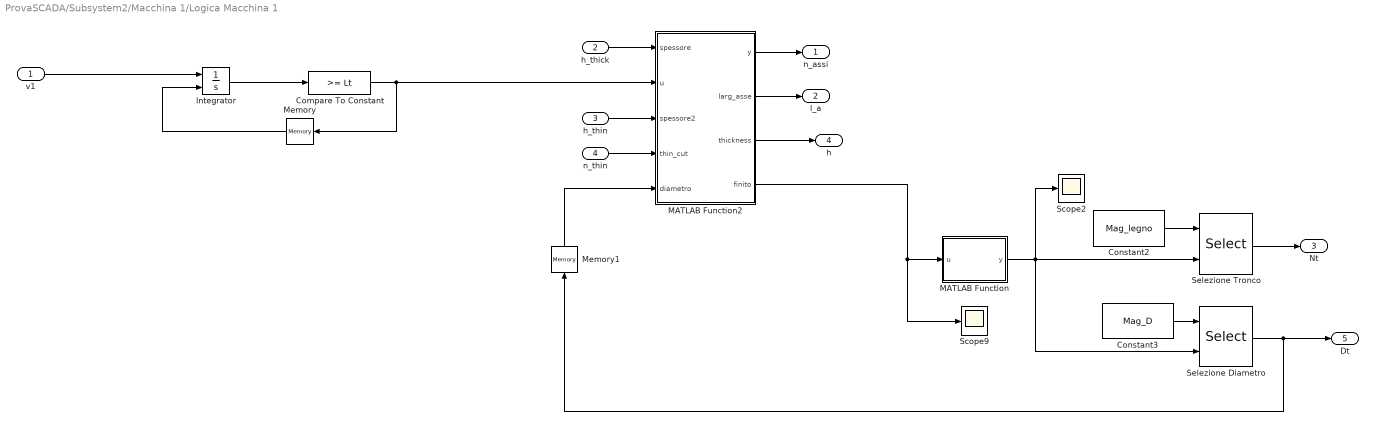
== system ProvaSCADA/Subsystem2/Macchina 1/Logica Macchina 1 ==
  v1 : Inport
  h_thick : Inport  Port=2
  h_thin : Inport  Port=3
  n_thin : Inport  Port=4
  Compare To Constant : simulink/Logic and Bit Operations/Compare To Constant  relop=>=  const=Lt  OutDataTypeStr=boolean
  Constant2 : Constant  Value=Mag_legno
  Constant3 : Constant  Value=Mag_D
  Integrator : Integrator  ExternalReset=rising
  MATLAB Function : MATLAB Function  TreatAsAtomicUnit=on
  MATLAB Function2 : MATLAB Function  TreatAsAtomicUnit=on
  Memory : Memory
  Memory1 : Memory
  Scope2 : Scope
  Scope9 : Scope
  Selezione Diametro : Selector  IndexMode=Zero-based  InputPortWidth=length(Mag_D)  IndexOptions=Index vector (port)  Indices=[1 3]  OutputSizes=1
  Selezione Tronco : Selector  IndexMode=Zero-based  InputPortWidth=length(Mag_legno)  IndexOptions=Index vector (port)  Indices=[1 3]  OutputSizes=1
  n_assi : Outport
  l_a : Outport  Port=2
  Nt : Outport  Port=3
  h : Outport  Port=4
  Dt : Outport  Port=5
  wires:
  Selezione Diametro/1 -> Dt/1, Memory1/1
  MATLAB Function2/4(finito) -> MATLAB Function/1(u), Scope9/1
  Memory/1 -> Integrator/2
  Memory1/1 -> MATLAB Function2/5(diametro)
  Constant2/1 -> Selezione Tronco/1
  v1/1 -> Integrator/1
  Integrator/1 -> Compare To Constant/1
  Constant3/1 -> Selezione Diametro/1
  MATLAB Function/1(y) -> Selezione Diametro/2, Scope2/1, Selezione Tronco/2
  MATLAB Function2/1(y) -> n_assi/1
  Selezione Tronco/1 -> Nt/1
  MATLAB Function2/2(larg_asse) -> l_a/1
  Compare To Constant/1 -> Memory/1, MATLAB Function2/2(u)
  h_thick/1 -> MATLAB Function2/1(spessore)
  h_thin/1 -> MATLAB Function2/3(spessore2)
  n_thin/1 -> MATLAB Function2/4(thin_cut)
  MATLAB Function2/3(thickness) -> h/1

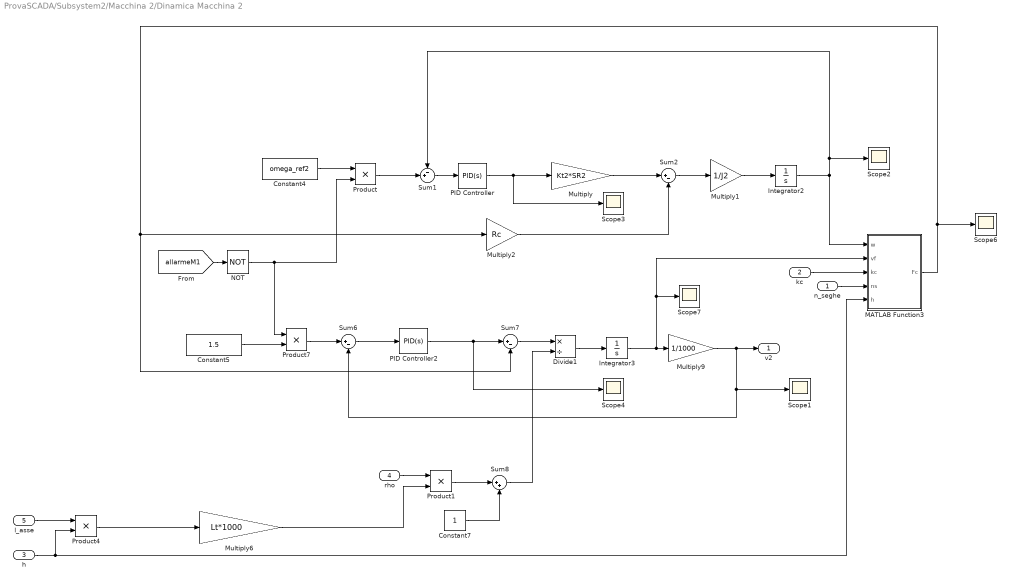
== system ProvaSCADA/Subsystem2/Macchina 2/Dinamica Macchina 2 ==
  n_seghe : Inport
  kc : Inport  Port=2
  h : Inport  Port=3
  rho : Inport  Port=4
  l_asse : Inport  Port=5
  Constant4 : Constant  Value=omega_ref2
  Constant5 : Constant  Value=1.5
  Constant7 : Constant
  Divide1 : Product  Inputs=*/
  Integrator2 : Integrator  InitialCondition=omega_ref2
  Integrator3 : Integrator  InitialCondition=1500
  MATLAB Function3 : MATLAB Function  TreatAsAtomicUnit=on
  Multiply : Gain  Gain=Kt2*SR2
  Multiply1 : Gain  Gain=1/J2
  Multiply2 : Gain  Gain=Rc
  Multiply6 : Gain  Gain=Lt*1000
  Multiply9 : Gain  Gain=1/1000
  NOT : Logic  Operator=NOT  IconShape=distinctive  AllPortsSameDT=off  OutDataTypeStr=boolean
  PID Controller : slpidlib/PID Controller  Controller=PID  Form=Parallel  TimeDomain=Continuous-time  UseExternalTs=off  SampleTime=-1  IntegratorMethod=Forward Euler  FilterMethod=Forward Euler  ControllerParametersSource=internal  P=345.484777327525  I=442.07289174245  UseKiTs=off  D=9.05690517196235  UseExternalDerivativeSource=off  N=26.4189049403583  UseFilter=on  TunerSelectOption=Transfer Function Based (PID Tuner App)  InitialConditionSource=internal  InitialConditionForIntegrator=0  InitialConditionForFilter=0  DifferentiatorICPrevScaledInput=0  ExternalReset=none  TrackingMode=off  Kt=1  LimitOutput=on  SatLimitsSource=internal  UpperSaturationLimit=300  LowerSaturationLimit=-300  LinearizeAsGain=on  AntiWindupMode=clamping  Kb=1  LimitIntegrator=off  UpperIntegratorSaturationLimit=200  LowerIntegratorSaturationLimit=-inf  POutMin=[]  POutMax=[]  IOutMin=[]  IOutMax=[]  DOutMin=[]  DOutMax=[]  NOutMin=[]  NOutMax=[]  SumOutMin=[]  SumOutMax=[]  SaturationOutMin=[]  SaturationOutMax=[]  PParamMin=[]  PParamMax=[]  IParamMin=[]  IParamMax=[]  DParamMin=[]  DParamMax=[]  NParamMin=[]  NParamMax=[]  KbParamMin=[]  KbParamMax=[]  KtParamMin=[]  KtParamMax=[]  KbOutMin=[]  KbOutMax=[]  KtOutMin=[]  KtOutMax=[]  IntegratorOutMin=[]  IntegratorOutMax=[]  FilterOutMin=[]  FilterOutMax=[]  SumI1OutMin=[]  SumI1OutMax=[]  SumI2OutMin=[]  SumI2OutMax=[]  SumI3OutMin=[]  SumI3OutMax=[]  SumI4OutMin=[]  SumI4OutMax=[]  SumDOutMin=[]  SumDOutMax=[]  DifferentiatorOutMin=[]  DifferentiatorOutMax=[]  FilterDiffOutCoefMin=[]  FilterDiffOutCoefMax=[]  ReciprocalOutMin=[]  ReciprocalOutMax=[]  SumDenOutMin=[]  SumDenOutMax=[]  SumNumOutMin=[]  SumNumOutMax=[]  DivideOutMin=[]  DivideOutMax=[]  UdiffTsProdOutMin=[]  UdiffTsProdOutMax=[]  NTsProdOutMin=[]  NTsProdOutMax=[]  UintegralTsProdOutMin=[]  UintegralTsProdOutMax=[]  UngainTsProdOutMin=[]  UngainTsProdOutMax=[]  ClampingZeroOutDataTypeStr=Inherit: Inherit via back propagation  ClampingZeroOutMin=[]  ClampingZeroOutMax=[]  FilterDenConstantOutDataTypeStr=Inherit: Inherit via back propagation  FilterDenConstantOutMin=[]  FilterDenConstantOutMax=[]  PCopyOutDataTypeStr=Inherit: Inherit via back propagation  PCopyOutMin=[]  PCopyOutMax=[]  NCopyOutDataTypeStr=Inherit: Inherit via back propagation  NCopyOutMin=[]  NCopyOutMax=[]  IntegratorContinuousStateAttributes=''  IntegratorStateMustResolveToSignalObject=off  IntegratorRTWStateStorageClass=Auto  FilterContinuousStateAttributes=''  FilterStateMustResolveToSignalObject=off  FilterRTWStateStorageClass=Auto  ParallelPVariant=InternalParameters  IdealPVariant=Disabled  IVariant=InternalParameters  DVariant=InternalParameters  IntegratorVariant=Continuous  SatVariant=Enabled  AWVariant=ContClampingParallel  PCopyVariant=Disabled  TRVariant=Disabled  FdbkBlocksVariant=Forward  IdealPFdbkVariant=Disabled  SatFdbkVariant=Disabled  DerivativeFilterVariant=ContFilter  NVariant=InternalParameters  NCopyVariant=Disabled  FilterICVariant=InternalICsFilter  IntegratorICVariant=InternalICs  ExternalResetVariant=Disabled  TRSumVariant=Passthrough  SumFdbkVariant=Disabled  SumVariant=Sum_PID  TsampFilterVariant=InternalTs  TsampNgainVariant=Passthrough  TsampIntegralVariant=Disabled_SignalSpec  ExternalSaturationOutDataTypeStr=Inherit: Same as second input  DerivativeSourceVariant=ErrorSignal  PreIntVariant=InternalPreInt
  PID Controller2 : slpidlib/PID Controller  Controller=PID  Form=Parallel  TimeDomain=Continuous-time  UseExternalTs=off  SampleTime=-1  IntegratorMethod=Forward Euler  FilterMethod=Forward Euler  ControllerParametersSource=internal  P=20866.9469532593  I=80635.0538109051  UseKiTs=off  D=181.138103439247  UseExternalDerivativeSource=off  N=79.7838174257724  UseFilter=on  TunerSelectOption=Transfer Function Based (PID Tuner App)  InitialConditionSource=internal  InitialConditionForIntegrator=0  InitialConditionForFilter=0  DifferentiatorICPrevScaledInput=0  ExternalReset=none  TrackingMode=off  Kt=1  LimitOutput=on  SatLimitsSource=internal  UpperSaturationLimit=5000  LowerSaturationLimit=-5000  LinearizeAsGain=off  AntiWindupMode=clamping  Kb=1  LimitIntegrator=off  UpperIntegratorSaturationLimit=200  LowerIntegratorSaturationLimit=-inf  POutMin=[]  POutMax=[]  IOutMin=[]  IOutMax=[]  DOutMin=[]  DOutMax=[]  NOutMin=[]  NOutMax=[]  SumOutMin=[]  SumOutMax=[]  SaturationOutMin=[]  SaturationOutMax=[]  PParamMin=[]  PParamMax=[]  IParamMin=[]  IParamMax=[]  DParamMin=[]  DParamMax=[]  NParamMin=[]  NParamMax=[]  KbParamMin=[]  KbParamMax=[]  KtParamMin=[]  KtParamMax=[]  KbOutMin=[]  KbOutMax=[]  KtOutMin=[]  KtOutMax=[]  IntegratorOutMin=[]  IntegratorOutMax=[]  FilterOutMin=[]  FilterOutMax=[]  SumI1OutMin=[]  SumI1OutMax=[]  SumI2OutMin=[]  SumI2OutMax=[]  SumI3OutMin=[]  SumI3OutMax=[]  SumI4OutMin=[]  SumI4OutMax=[]  SumDOutMin=[]  SumDOutMax=[]  DifferentiatorOutMin=[]  DifferentiatorOutMax=[]  FilterDiffOutCoefMin=[]  FilterDiffOutCoefMax=[]  ReciprocalOutMin=[]  ReciprocalOutMax=[]  SumDenOutMin=[]  SumDenOutMax=[]  SumNumOutMin=[]  SumNumOutMax=[]  DivideOutMin=[]  DivideOutMax=[]  UdiffTsProdOutMin=[]  UdiffTsProdOutMax=[]  NTsProdOutMin=[]  NTsProdOutMax=[]  UintegralTsProdOutMin=[]  UintegralTsProdOutMax=[]  UngainTsProdOutMin=[]  UngainTsProdOutMax=[]  ClampingZeroOutDataTypeStr=Inherit: Inherit via back propagation  ClampingZeroOutMin=[]  ClampingZeroOutMax=[]  FilterDenConstantOutDataTypeStr=Inherit: Inherit via back propagation  FilterDenConstantOutMin=[]  FilterDenConstantOutMax=[]  PCopyOutDataTypeStr=Inherit: Inherit via back propagation  PCopyOutMin=[]  PCopyOutMax=[]  NCopyOutDataTypeStr=Inherit: Inherit via back propagation  NCopyOutMin=[]  NCopyOutMax=[]  IntegratorContinuousStateAttributes=''  IntegratorStateMustResolveToSignalObject=off  IntegratorRTWStateStorageClass=Auto  FilterContinuousStateAttributes=''  FilterStateMustResolveToSignalObject=off  FilterRTWStateStorageClass=Auto  ParallelPVariant=InternalParameters  IdealPVariant=Disabled  IVariant=InternalParameters  DVariant=InternalParameters  IntegratorVariant=Continuous  SatVariant=Enabled  AWVariant=ContClampingParallel  PCopyVariant=Disabled  TRVariant=Disabled  FdbkBlocksVariant=Forward  IdealPFdbkVariant=Disabled  SatFdbkVariant=Disabled  DerivativeFilterVariant=ContFilter  NVariant=InternalParameters  NCopyVariant=Disabled  FilterICVariant=InternalICsFilter  IntegratorICVariant=InternalICs  ExternalResetVariant=Disabled  TRSumVariant=Passthrough  SumFdbkVariant=Disabled  SumVariant=Sum_PID  TsampFilterVariant=InternalTs  TsampNgainVariant=Passthrough  TsampIntegralVariant=Disabled_SignalSpec  ExternalSaturationOutDataTypeStr=Inherit: Same as second input  DerivativeSourceVariant=ErrorSignal  PreIntVariant=InternalPreInt
  Product{,1,4,7} (4 alike) : Product
  Scope{1..4,6..7} (6 alike) : Scope
  Sum1 : Sum  Inputs=-+|
  Sum2 : Sum  Inputs=|+-
  Sum6 : Sum  Inputs=|+-
  Sum7 : Sum  Inputs=|+-
  Sum8 : Sum  Inputs=|++
  v2 : Outport
  wires:
  Product4/1 -> Multiply6/1
  h/1 -> MATLAB Function3/5(h), Product4/2
  l_asse/1 -> Product4/1
  Constant4/1 -> Product/1
  Constant5/1 -> Product7/2
  Product/1 -> Sum1/2
  Sum1/1 -> PID Controller/1
  rho/1 -> Product1/1
  NOT/1 -> Product/2, Product7/1
  Multiply1/1 -> Integrator2/1
  PID Controller/1 -> Scope3/1, Multiply/1
  MATLAB Function3/1(Fc) -> Multiply2/1, Sum7/2, Scope6/1
  Sum6/1 -> PID Controller2/1
  Divide1/1 -> Integrator3/1
  Integrator3/1 -> Scope7/1, MATLAB Function3/2(vf), Multiply9/1
  PID Controller2/1 -> Sum7/1, Scope4/1
  Integrator2/1 -> MATLAB Function3/1(w), Scope2/1, Sum1/1
  Sum7/1 -> Divide1/1
  Product7/1 -> Sum6/1
  kc/1 -> MATLAB Function3/3(kc)
  Multiply6/1 -> Product1/2
  n_seghe/1 -> MATLAB Function3/4(ns)
  Product1/1 -> Sum8/1
  Sum8/1 -> Divide1/2
  Constant7/1 -> Sum8/2
  Multiply9/1 -> v2/1, Scope1/1, Sum6/2
  [allarmeM1] -> NOT/1
  Multiply/1 -> Sum2/1
  Sum2/1 -> Multiply1/1
  Multiply2/1 -> Sum2/2

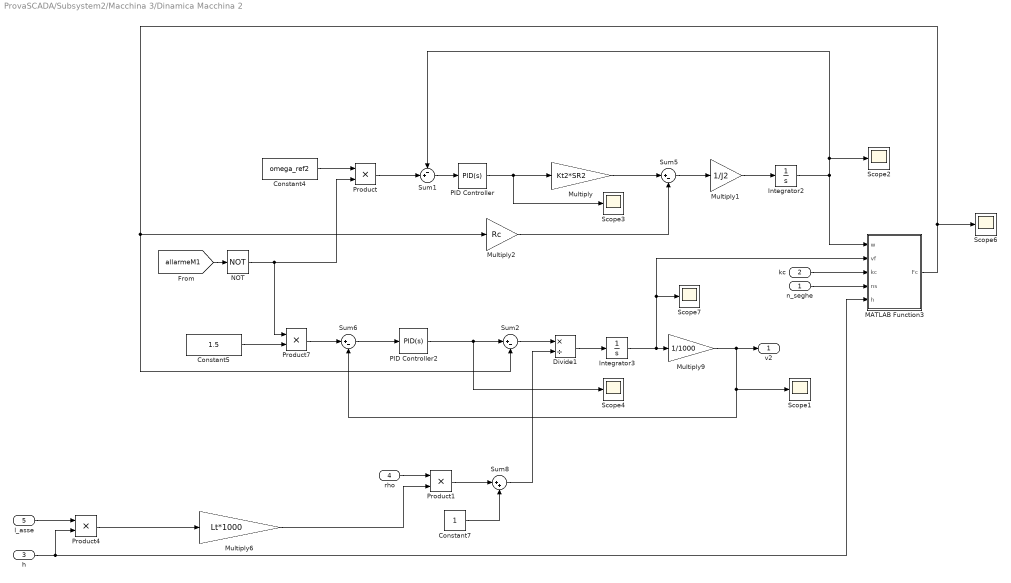
== system ProvaSCADA/Subsystem2/Macchina 3/Dinamica Macchina 2 ==
  n_seghe : Inport
  kc : Inport  Port=2
  h : Inport  Port=3
  rho : Inport  Port=4
  l_asse : Inport  Port=5
  Constant4 : Constant  Value=omega_ref2
  Constant5 : Constant  Value=1.5
  Constant7 : Constant
  Divide1 : Product  Inputs=*/
  Integrator2 : Integrator  InitialCondition=omega_ref2
  Integrator3 : Integrator  InitialCondition=1500
  MATLAB Function3 : MATLAB Function  TreatAsAtomicUnit=on
  Multiply : Gain  Gain=Kt2*SR2
  Multiply1 : Gain  Gain=1/J2
  Multiply2 : Gain  Gain=Rc
  Multiply6 : Gain  Gain=Lt*1000
  Multiply9 : Gain  Gain=1/1000
  NOT : Logic  Operator=NOT  IconShape=distinctive  AllPortsSameDT=off  OutDataTypeStr=boolean
  PID Controller : slpidlib/PID Controller  Controller=PID  Form=Parallel  TimeDomain=Continuous-time  UseExternalTs=off  SampleTime=-1  IntegratorMethod=Forward Euler  FilterMethod=Forward Euler  ControllerParametersSource=internal  P=345.484777327525  I=442.07289174245  UseKiTs=off  D=9.05690517196235  UseExternalDerivativeSource=off  N=26.4189049403583  UseFilter=on  TunerSelectOption=Transfer Function Based (PID Tuner App)  InitialConditionSource=internal  InitialConditionForIntegrator=0  InitialConditionForFilter=0  DifferentiatorICPrevScaledInput=0  ExternalReset=none  TrackingMode=off  Kt=1  LimitOutput=on  SatLimitsSource=internal  UpperSaturationLimit=300  LowerSaturationLimit=-300  LinearizeAsGain=on  AntiWindupMode=clamping  Kb=1  LimitIntegrator=off  UpperIntegratorSaturationLimit=200  LowerIntegratorSaturationLimit=-inf  POutMin=[]  POutMax=[]  IOutMin=[]  IOutMax=[]  DOutMin=[]  DOutMax=[]  NOutMin=[]  NOutMax=[]  SumOutMin=[]  SumOutMax=[]  SaturationOutMin=[]  SaturationOutMax=[]  PParamMin=[]  PParamMax=[]  IParamMin=[]  IParamMax=[]  DParamMin=[]  DParamMax=[]  NParamMin=[]  NParamMax=[]  KbParamMin=[]  KbParamMax=[]  KtParamMin=[]  KtParamMax=[]  KbOutMin=[]  KbOutMax=[]  KtOutMin=[]  KtOutMax=[]  IntegratorOutMin=[]  IntegratorOutMax=[]  FilterOutMin=[]  FilterOutMax=[]  SumI1OutMin=[]  SumI1OutMax=[]  SumI2OutMin=[]  SumI2OutMax=[]  SumI3OutMin=[]  SumI3OutMax=[]  SumI4OutMin=[]  SumI4OutMax=[]  SumDOutMin=[]  SumDOutMax=[]  DifferentiatorOutMin=[]  DifferentiatorOutMax=[]  FilterDiffOutCoefMin=[]  FilterDiffOutCoefMax=[]  ReciprocalOutMin=[]  ReciprocalOutMax=[]  SumDenOutMin=[]  SumDenOutMax=[]  SumNumOutMin=[]  SumNumOutMax=[]  DivideOutMin=[]  DivideOutMax=[]  UdiffTsProdOutMin=[]  UdiffTsProdOutMax=[]  NTsProdOutMin=[]  NTsProdOutMax=[]  UintegralTsProdOutMin=[]  UintegralTsProdOutMax=[]  UngainTsProdOutMin=[]  UngainTsProdOutMax=[]  ClampingZeroOutDataTypeStr=Inherit: Inherit via back propagation  ClampingZeroOutMin=[]  ClampingZeroOutMax=[]  FilterDenConstantOutDataTypeStr=Inherit: Inherit via back propagation  FilterDenConstantOutMin=[]  FilterDenConstantOutMax=[]  PCopyOutDataTypeStr=Inherit: Inherit via back propagation  PCopyOutMin=[]  PCopyOutMax=[]  NCopyOutDataTypeStr=Inherit: Inherit via back propagation  NCopyOutMin=[]  NCopyOutMax=[]  IntegratorContinuousStateAttributes=''  IntegratorStateMustResolveToSignalObject=off  IntegratorRTWStateStorageClass=Auto  FilterContinuousStateAttributes=''  FilterStateMustResolveToSignalObject=off  FilterRTWStateStorageClass=Auto  ParallelPVariant=InternalParameters  IdealPVariant=Disabled  IVariant=InternalParameters  DVariant=InternalParameters  IntegratorVariant=Continuous  SatVariant=Enabled  AWVariant=ContClampingParallel  PCopyVariant=Disabled  TRVariant=Disabled  FdbkBlocksVariant=Forward  IdealPFdbkVariant=Disabled  SatFdbkVariant=Disabled  DerivativeFilterVariant=ContFilter  NVariant=InternalParameters  NCopyVariant=Disabled  FilterICVariant=InternalICsFilter  IntegratorICVariant=InternalICs  ExternalResetVariant=Disabled  TRSumVariant=Passthrough  SumFdbkVariant=Disabled  SumVariant=Sum_PID  TsampFilterVariant=InternalTs  TsampNgainVariant=Passthrough  TsampIntegralVariant=Disabled_SignalSpec  ExternalSaturationOutDataTypeStr=Inherit: Same as second input  DerivativeSourceVariant=ErrorSignal  PreIntVariant=InternalPreInt
  PID Controller2 : slpidlib/PID Controller  Controller=PID  Form=Parallel  TimeDomain=Continuous-time  UseExternalTs=off  SampleTime=-1  IntegratorMethod=Forward Euler  FilterMethod=Forward Euler  ControllerParametersSource=internal  P=20866.9469532593  I=80635.0538109051  UseKiTs=off  D=181.138103439247  UseExternalDerivativeSource=off  N=79.7838174257724  UseFilter=on  TunerSelectOption=Transfer Function Based (PID Tuner App)  InitialConditionSource=internal  InitialConditionForIntegrator=0  InitialConditionForFilter=0  DifferentiatorICPrevScaledInput=0  ExternalReset=none  TrackingMode=off  Kt=1  LimitOutput=on  SatLimitsSource=internal  UpperSaturationLimit=5000  LowerSaturationLimit=-5000  LinearizeAsGain=off  AntiWindupMode=clamping  Kb=1  LimitIntegrator=off  UpperIntegratorSaturationLimit=200  LowerIntegratorSaturationLimit=-inf  POutMin=[]  POutMax=[]  IOutMin=[]  IOutMax=[]  DOutMin=[]  DOutMax=[]  NOutMin=[]  NOutMax=[]  SumOutMin=[]  SumOutMax=[]  SaturationOutMin=[]  SaturationOutMax=[]  PParamMin=[]  PParamMax=[]  IParamMin=[]  IParamMax=[]  DParamMin=[]  DParamMax=[]  NParamMin=[]  NParamMax=[]  KbParamMin=[]  KbParamMax=[]  KtParamMin=[]  KtParamMax=[]  KbOutMin=[]  KbOutMax=[]  KtOutMin=[]  KtOutMax=[]  IntegratorOutMin=[]  IntegratorOutMax=[]  FilterOutMin=[]  FilterOutMax=[]  SumI1OutMin=[]  SumI1OutMax=[]  SumI2OutMin=[]  SumI2OutMax=[]  SumI3OutMin=[]  SumI3OutMax=[]  SumI4OutMin=[]  SumI4OutMax=[]  SumDOutMin=[]  SumDOutMax=[]  DifferentiatorOutMin=[]  DifferentiatorOutMax=[]  FilterDiffOutCoefMin=[]  FilterDiffOutCoefMax=[]  ReciprocalOutMin=[]  ReciprocalOutMax=[]  SumDenOutMin=[]  SumDenOutMax=[]  SumNumOutMin=[]  SumNumOutMax=[]  DivideOutMin=[]  DivideOutMax=[]  UdiffTsProdOutMin=[]  UdiffTsProdOutMax=[]  NTsProdOutMin=[]  NTsProdOutMax=[]  UintegralTsProdOutMin=[]  UintegralTsProdOutMax=[]  UngainTsProdOutMin=[]  UngainTsProdOutMax=[]  ClampingZeroOutDataTypeStr=Inherit: Inherit via back propagation  ClampingZeroOutMin=[]  ClampingZeroOutMax=[]  FilterDenConstantOutDataTypeStr=Inherit: Inherit via back propagation  FilterDenConstantOutMin=[]  FilterDenConstantOutMax=[]  PCopyOutDataTypeStr=Inherit: Inherit via back propagation  PCopyOutMin=[]  PCopyOutMax=[]  NCopyOutDataTypeStr=Inherit: Inherit via back propagation  NCopyOutMin=[]  NCopyOutMax=[]  IntegratorContinuousStateAttributes=''  IntegratorStateMustResolveToSignalObject=off  IntegratorRTWStateStorageClass=Auto  FilterContinuousStateAttributes=''  FilterStateMustResolveToSignalObject=off  FilterRTWStateStorageClass=Auto  ParallelPVariant=InternalParameters  IdealPVariant=Disabled  IVariant=InternalParameters  DVariant=InternalParameters  IntegratorVariant=Continuous  SatVariant=Enabled  AWVariant=ContClampingParallel  PCopyVariant=Disabled  TRVariant=Disabled  FdbkBlocksVariant=Forward  IdealPFdbkVariant=Disabled  SatFdbkVariant=Disabled  DerivativeFilterVariant=ContFilter  NVariant=InternalParameters  NCopyVariant=Disabled  FilterICVariant=InternalICsFilter  IntegratorICVariant=InternalICs  ExternalResetVariant=Disabled  TRSumVariant=Passthrough  SumFdbkVariant=Disabled  SumVariant=Sum_PID  TsampFilterVariant=InternalTs  TsampNgainVariant=Passthrough  TsampIntegralVariant=Disabled_SignalSpec  ExternalSaturationOutDataTypeStr=Inherit: Same as second input  DerivativeSourceVariant=ErrorSignal  PreIntVariant=InternalPreInt
  Product{,1,4,7} (4 alike) : Product
  Scope{1..4,6..7} (6 alike) : Scope
  Sum1 : Sum  Inputs=-+|
  Sum2 : Sum  Inputs=|+-
  Sum5 : Sum  Inputs=|+-
  Sum6 : Sum  Inputs=|+-
  Sum8 : Sum  Inputs=|++
  v2 : Outport
  wires:
  Product4/1 -> Multiply6/1
  h/1 -> MATLAB Function3/5(h), Product4/2
  l_asse/1 -> Product4/1
  Constant4/1 -> Product/1
  Constant5/1 -> Product7/2
  Product/1 -> Sum1/2
  Sum1/1 -> PID Controller/1
  rho/1 -> Product1/1
  NOT/1 -> Product/2, Product7/1
  Sum5/1 -> Multiply1/1
  Multiply1/1 -> Integrator2/1
  PID Controller/1 -> Scope3/1, Multiply/1
  MATLAB Function3/1(Fc) -> Sum2/2, Multiply2/1, Scope6/1
  Sum6/1 -> PID Controller2/1
  Divide1/1 -> Integrator3/1
  Integrator3/1 -> Scope7/1, MATLAB Function3/2(vf), Multiply9/1
  PID Controller2/1 -> Sum2/1, Scope4/1
  Integrator2/1 -> MATLAB Function3/1(w), Scope2/1, Sum1/1
  Sum2/1 -> Divide1/1
  Product7/1 -> Sum6/1
  kc/1 -> MATLAB Function3/3(kc)
  Multiply6/1 -> Product1/2
  n_seghe/1 -> MATLAB Function3/4(ns)
  Product1/1 -> Sum8/1
  Sum8/1 -> Divide1/2
  Constant7/1 -> Sum8/2
  Multiply9/1 -> v2/1, Scope1/1, Sum6/2
  [allarmeM1] -> NOT/1
  Multiply/1 -> Sum5/1
  Multiply2/1 -> Sum5/2

== matlab function ProvaSCADA/Subsystem2/MATLAB Function1 ==
  data: u input; y output
function y = fcn(u)

    persistent n_prec

    if isempty(n_prec)
        n_prec = 0;
    end

    y = u - n_prec;

    n_prec = u;

== matlab function ProvaSCADA/Subsystem1/MATLAB Function4 ==
  data: u input; idx output; h_index parameter
function idx = find_index(u, h_index)
%#codegen

v = h_index;

idx = -1; % valore default se non trovato

for i = 1:length(v)
    if u == v(i)
        idx = i;
        return;
    end
end

== matlab function ProvaSCADA/Subsystem1/MATLAB Function5 ==
  data: u input; idx output; l_index parameter
function idx = find_index(u, l_index)
%#codegen

v = l_index;

idx = -1; % valore default se non trovato

for i = 1:length(v)
    if u == v(i)
        idx = i;
        return;
    end
end

== matlab function ProvaSCADA/Subsystem2/Macchina 2/Dinamica Macchina 2/MATLAB Function3 ==
  data: w input; Fc output; vf input; kc input; ns input; h input; Rs parameter; b parameter
function Fc = Fcfun(w, vf, kc, ns, h, Rs, b)

if w < 0.01
    Fc = 0;
else
    Fc = ns*kc*b*vf*h/(w*Rs);
end

== matlab function ProvaSCADA/Subsystem2/Macchina 3/Dinamica Macchina 2/MATLAB Function3 ==
  data: w input; Fc output; vf input; kc input; ns input; h input; Rs parameter; b parameter
function Fc = Fcfun(w, vf, kc, ns, h, Rs, b)

if w < 0.01
    Fc = 0;
else
    Fc = ns*kc*b*vf*h/(w*Rs);
end

== matlab function ProvaSCADA/Subsystem2/Macchina 3/MATLAB Function2 ==
  settings: updateMethod=DISCRETE
  data: u input; w_asse input; y output; l_asse input; taglio output; Lt parameter
function [y, taglio] = fcn(u, w_asse, l_asse,Lt)
    persistent counter 

    n_assi = floor(l_asse / w_asse);
    
    taglio = 0;

    if isempty(counter)
        counter = 0;
    end

    % Conto assi tagliate
    if u >= Lt
        counter = counter + n_assi;
    end

    % Segnale di taglio
    if  (u > 0 && u < Lt && l_asse > 0) 
        taglio = 1;
    end
    y = counter;
end

== matlab function ProvaSCADA/Subsystem2/Macchina 2/MATLAB Function2 ==
  settings: updateMethod=DISCRETE
  data: u input; w_asse input; y output; l_asse input; taglio output; Lt parameter
function [y, taglio] = fcn(u, w_asse, l_asse,Lt)
    persistent counter 

    n_assi = floor(l_asse / w_asse);
    
    taglio = 0;

    if isempty(counter)
        counter = 0;
    end

    % Conto assi tagliate
    if u >= Lt
        counter = counter + n_assi;
    end

    % Segnale di taglio
    if  (u > 0 && u < Lt && l_asse > 0) 
        taglio = 1;
    end
    y = counter;
end

== matlab function ProvaSCADA/Subsystem2/Macchina 1/Logica Macchina 1/MATLAB Function ==
  data: u input; y output; Mag_legno parameter
function y = fcn(u, Mag_legno)
    persistent counter
    if isempty(counter)
        counter = 1;
    end

    if u == 1
        counter = counter + 1;
    end

    y = counter;
    
    if y > length(Mag_legno)-1
        y = 0;
    end

end

== matlab function ProvaSCADA/Subsystem2/Macchina 1/Logica Macchina 1/MATLAB Function2 ==
  settings: updateMethod=DISCRETE
  data: spessore input; u input; spessore2 input; thin_cut input; diametro input; y output; larg_asse output; thickness output; finito output
function [y, larg_asse, thickness, finito]= fcn(spessore, u, spessore2, thin_cut, diametro)
    persistent counter 

  
    max_assi = floor((diametro-thin_cut*spessore2) / spessore);
    finito = 0;
    
    if isempty(counter)
        counter = 0;
    end

    % Conto assi tagliate
    if u == 1
        counter = counter + 1;
    end

    % Quando finisco tronco segnalo e azzero counter
    if counter > max_assi + thin_cut
        finito = 1;
        counter = 0;
    end

    
    if counter == 0
        larg_asse = 0;
        thickness = 0;
    elseif counter <= thin_cut/2
        distanza_bordo = counter * spessore2;
        h = abs(diametro/2 - distanza_bordo + (spessore2/2));
        larg_asse = 2 * sqrt((diametro/2)^2-h^2);
        thickness = spessore2;
    elseif counter > max_assi + thin_cut/2
        distanza_bordo = max_assi*spessore + (counter-max_assi)*spessore2;
        h = abs(diametro/2 - distanza_bordo + (spessore2/2));
        larg_asse = 2 * sqrt((diametro/2)^2-h^2);
        thickness = spessore2;
    else
        % Calcolo larghezza delle assi
        distanza_bordo = thin_cut/2 * spessore2 + (counter-thin_cut/2) * spessore;
        h = abs(diametro/2 - distanza_bordo + (spessore/2));
        larg_asse = 2 * sqrt((diametro/2)^2-h^2);
        thickness = spessore;
    end
    

    y = counter;

== matlab function ProvaSCADA/Subsystem2/Macchina 1/Dinamica Macchina 1/MATLAB Function3 ==
  data: w input; Fc output; vf input; kc input; Dt input; Rs parameter; b parameter
function Fc = Fcfun(w, vf, kc, Dt, Rs, b)

if w < 0.01
    Fc = 0;
else
    Fc = kc*b*vf*Dt/(w*Rs);
end

== matlab function ProvaSCADA/Subsystem2/MATLAB Function ==
  data: u input; y output
function y = fcn(u)

    persistent n_prec

    if isempty(n_prec)
        n_prec = 0;
    end

    y = u - n_prec;


    n_prec = u;

== matlab function ProvaSCADA/Subsystem1/MATLAB Function1 ==
  data: u input; idx output; h_index parameter
function idx = find_index(u, h_index)
%#codegen

v = h_index;

idx = -1; % valore default se non trovato

for i = 1:length(v)
    if u == v(i)
        idx = i;
        return;
    end
end

== matlab function ProvaSCADA/Subsystem1/MATLAB Function2 ==
  data: u input; idx output; l_index parameter
function idx = find_index(u, l_index)
%#codegen

v = l_index;

idx = -1; % valore default se non trovato

for i = 1:length(v)
    if u == v(i)
        idx = i;
        return;
    end
end
